simulink model "GameModel"  (R2024a)
settings: Solver=VariableStepAuto  StartTime=0.0  StopTime=inf  MaxStep=0.02  RelTol=1e-3
model workspace (MAT data in the model file):
  g = 9.81
undefined symbols (not defined in the file or in its folder): CR, LF
libraries: simulink x8, instrumentseriallib x2
settings Model: Creator=Admin  LastModifiedBy=Michael Scopchanov

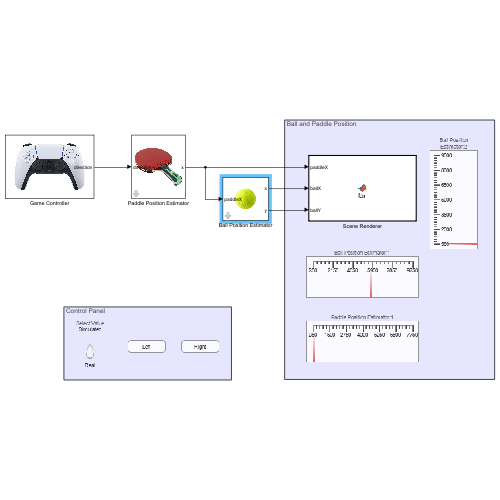
[thumbnail: Simulink's stored preview of the top-level diagram]
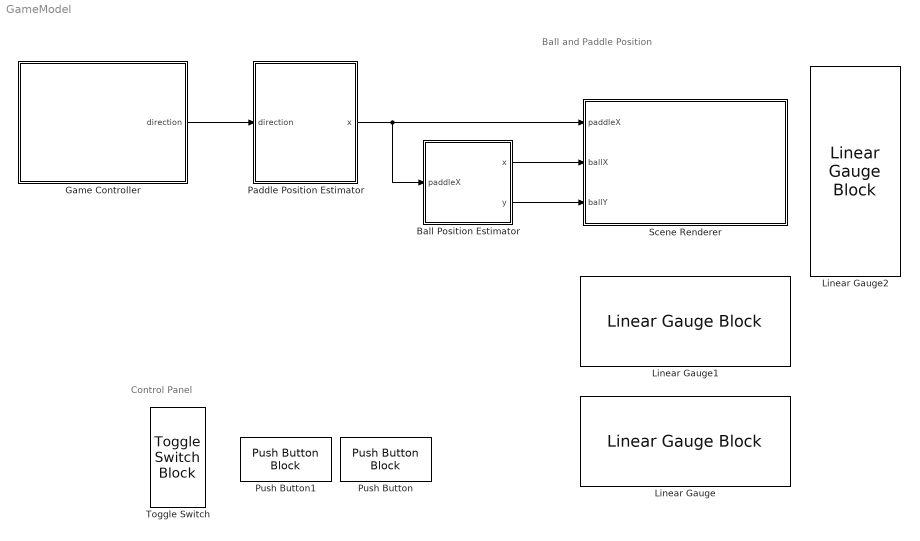
== system GameModel ==
  note: Ball and Paddle Position
  note: Control Panel
  Ball Position Estimator : Subsystem  mask{m=0.05, x0=4875, y0=4000, vn=10000}
      mask prompts: m "Mass [kg]"; x0 "Initial Position x [m]"; y0 "Initial Position y [m]"; vn "Nominal velocity [m/s]"
      mask Display: image('ball.png', [20,20,20,20,100,100]);
  Game Controller : Subsystem
      mask Display: image('controller.png', [10,10,10,10,100,100]);
  Linear Gauge : LinearGaugeBlock  ScaleMin=250  ScaleMax=7750
  Linear Gauge1 : LinearGaugeBlock  ScaleMin=250  ScaleMax=9750
  Linear Gauge2 : LinearGaugeBlock  ScaleMin=500  ScaleMax=9500
  Paddle Position Estimator : Subsystem  mask(Paddle Position Estimator){vn=15000, x0=4000, xmin=250, xmax=7750}
      mask prompts: vn "Nominal velocity [m/s]"; x0 "Initial position [m]"; xmin "Minimal position [m]"; xmax "Maximum position [m]"
      mask Display: image('paddle.jpg');
  Push Button : PushButtonBlock  ButtonText=Right  OnValue=0  OffValue=1.000000
  Push Button1 : PushButtonBlock  ButtonText=Left  OnValue=0  OffValue=1.000000
  Scene Renderer : MATLAB Function  InitFcn=handles = setupGraphics();  TreatAsAtomicUnit=on
  Toggle Switch : ToggleSwitchBlock
      settings: Values={{'Real', 'Simulated'}, [0 1]}
  wires:
  Game Controller/1(direction) -> Paddle Position Estimator/1(direction)
  Ball Position Estimator/1(x) -> Scene Renderer/2(ballX)
  Ball Position Estimator/2(y) -> Scene Renderer/3(ballY)
  Paddle Position Estimator/1(x) -> Ball Position Estimator/1(paddleX), Scene Renderer/1(paddleX)

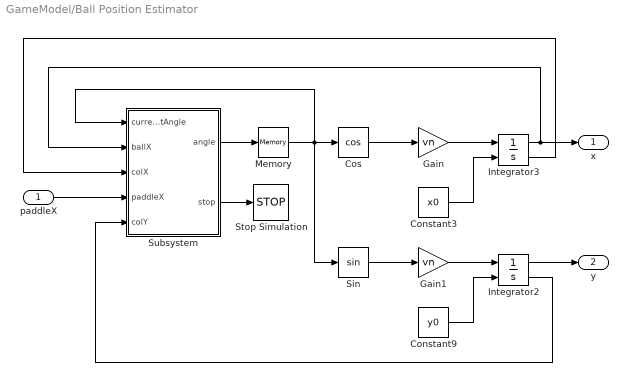
== system GameModel/Ball Position Estimator ==
  paddleX : Inport
  Constant3 : Constant  Value=x0
  Constant9 : Constant  Value=y0
  Cos : Trigonometry  Operator=cos
  Gain : Gain  Gain=vn
  Gain1 : Gain  Gain=vn
  Integrator2 : Integrator  InitialConditionSource=external  LimitOutput=on  UpperSaturationLimit=9500  LowerSaturationLimit=500  ShowSaturationPort=on
  Integrator3 : Integrator  InitialConditionSource=external  LimitOutput=on  UpperSaturationLimit=9500  LowerSaturationLimit=250  ShowSaturationPort=on
  Memory : Memory  InitialCondition=pi/3
  Sin : Trigonometry
  Stop Simulation : Stop
  Subsystem : Subsystem
  x : Outport
  y : Outport  Port=2
  wires:
  Integrator3/1 -> x/1, Subsystem/2(ballX)
  Constant3/1 -> Integrator3/2
  Integrator3/2 -> Subsystem/3(colX)
  Integrator2/2 -> Subsystem/5(colY)
  Constant9/1 -> Integrator2/2
  Integrator2/1 -> y/1
  Sin/1 -> Gain1/1
  Cos/1 -> Gain/1
  Memory/1 -> Subsystem/1(currentAngle), Sin/1, Cos/1
  Subsystem/1(angle) -> Memory/1
  paddleX/1 -> Subsystem/4(paddleX)
  Gain/1 -> Integrator3/1
  Gain1/1 -> Integrator2/1
  Subsystem/2(stop) -> Stop Simulation/1

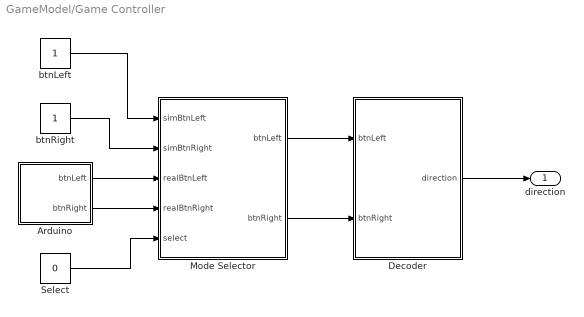
== system GameModel/Game Controller ==
  Arduino : Subsystem
      mask Display: image('arduino.jpg');
  Decoder : Subsystem
  Mode Selector : Subsystem
  Select : Constant  Value=0
  btnLeft : Constant
  btnRight : Constant
  direction : Outport
  wires:
  Arduino/2(btnRight) -> Mode Selector/4(realBtnRight)
  btnRight/1 -> Mode Selector/2(simBtnRight)
  Mode Selector/1(btnLeft) -> Decoder/1(btnLeft)
  Mode Selector/2(btnRight) -> Decoder/2(btnRight)
  btnLeft/1 -> Mode Selector/1(simBtnLeft)
  Decoder/1(direction) -> direction/1
  Select/1 -> Mode Selector/5(select)
  Arduino/1(btnLeft) -> Mode Selector/3(realBtnLeft)

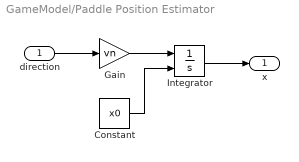
== system GameModel/Paddle Position Estimator ==
  direction : Inport
  Constant : Constant  Value=x0
  Gain : Gain  Gain=vn
  Integrator : Integrator  InitialConditionSource=external  LimitOutput=on  UpperSaturationLimit=xmax  LowerSaturationLimit=xmin
  x : Outport
  wires:
  direction/1 -> Gain/1
  Gain/1 -> Integrator/1
  Integrator/1 -> x/1
  Constant/1 -> Integrator/2

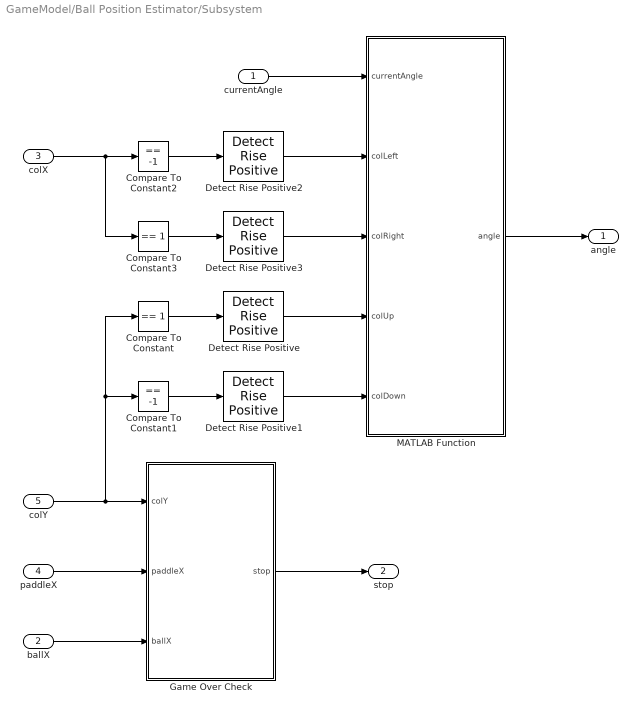
== system GameModel/Ball Position Estimator/Subsystem ==
  currentAngle : Inport
  ballX : Inport  Port=2
  colX : Inport  Port=3
  paddleX : Inport  Port=4
  colY : Inport  Port=5
  Compare To Constant : simulink/Logic and Bit Operations/Compare To Constant  relop===  const=1  OutDataTypeStr=boolean
  Compare To Constant1 : simulink/Logic and Bit Operations/Compare To Constant  relop===  const=-1  OutDataTypeStr=boolean
  Compare To Constant2 : simulink/Logic and Bit Operations/Compare To Constant  relop===  const=-1  OutDataTypeStr=boolean
  Compare To Constant3 : simulink/Logic and Bit Operations/Compare To Constant  relop===  const=1  OutDataTypeStr=boolean
  Detect Rise Positive{,1..3} (4 alike) : simulink/Logic and Bit Operations/Detect Rise Positive  vinit=0  OutDataTypeStr=boolean
  Game Over Check : MATLAB Function  TreatAsAtomicUnit=on
  MATLAB Function : MATLAB Function  TreatAsAtomicUnit=on
  angle : Outport
  stop : Outport  Port=2
  wires:
  MATLAB Function/1(angle) -> angle/1
  colY/1 -> Game Over Check/1(colY), Compare To Constant/1, Compare To Constant1/1
  paddleX/1 -> Game Over Check/2(paddleX)
  ballX/1 -> Game Over Check/3(ballX)
  Game Over Check/1(stop) -> stop/1
  currentAngle/1 -> MATLAB Function/1(currentAngle)
  colX/1 -> Compare To Constant3/1, Compare To Constant2/1
  Compare To Constant/1 -> Detect Rise Positive/1
  Detect Rise Positive/1 -> MATLAB Function/4(colUp)
  Compare To Constant1/1 -> Detect Rise Positive1/1
  Detect Rise Positive1/1 -> MATLAB Function/5(colDown)
  Compare To Constant2/1 -> Detect Rise Positive2/1
  Detect Rise Positive2/1 -> MATLAB Function/2(colLeft)
  Compare To Constant3/1 -> Detect Rise Positive3/1
  Detect Rise Positive3/1 -> MATLAB Function/3(colRight)

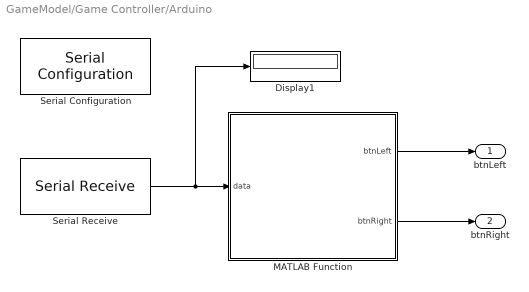
== system GameModel/Game Controller/Arduino ==
  Display1 : Display
  MATLAB Function : MATLAB Function  TreatAsAtomicUnit=on
  Serial Configuration : instrumentseriallib/Serial Configuration  Priority=-200000  PortSel=COM3  Port=COM3  ComPort=COM3  BaudRate=19200  DataBits=8  Parity=none  StopBits=1  ByteOrder=little-endian  FlowControl=none  Timeout=10  SimulateUsing=Interpreted execution  BlockInModel=on  aMode=1
  Serial Receive : instrumentseriallib/Serial Receive  Priority=1  PortSel=COM3  Port=COM3  ComPort=COM3  DataType=uint8  SaveDataType=uint8  ToggleHeader=off  Header=[]  ToggleDataSize=on  DataSize=[1 1]  ToggleTerminator=off  Terminator=CR/LF ('\r\n')  CustomTerminator=[]  InputFormat=Column major  EnableBlockingMode=on  ActionDataUnavailable=Output custom value  ActionWhenDataUnavailable=Output custom value  CustomValue=0  SampleTime=0.01  SimulateUsing=Interpreted execution  BlockInModel=on  aMode=1
  btnLeft : Outport
  btnRight : Outport  Port=2
  wires:
  MATLAB Function/1(btnLeft) -> btnLeft/1
  MATLAB Function/2(btnRight) -> btnRight/1
  Serial Receive/1 -> Display1/1, MATLAB Function/1(data)

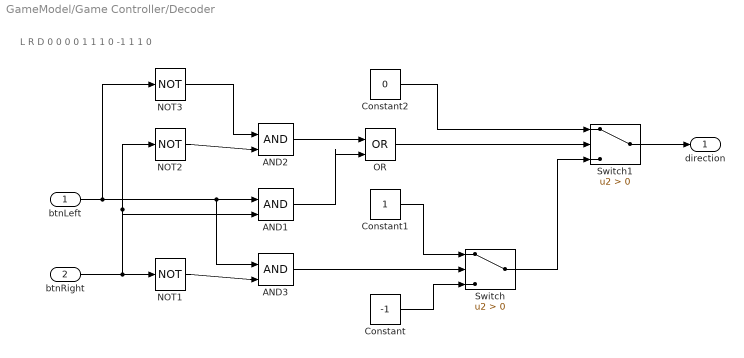
== system GameModel/Game Controller/Decoder ==
  note: L
      | R
      | D
      |
      | 0
      | 0
      | 0
      |
      | 0
      | 1
      | 1
      |
      | 1
      | 0
      | -1
      |
      | 1
      | 1
      | 0
  btnLeft : Inport
  btnRight : Inport  Port=2
  AND1 : Logic  IconShape=distinctive  AllPortsSameDT=off  OutDataTypeStr=boolean
  AND2 : Logic  IconShape=distinctive  AllPortsSameDT=off  OutDataTypeStr=boolean
  AND3 : Logic  IconShape=distinctive  AllPortsSameDT=off  OutDataTypeStr=boolean
  Constant : Constant  Value=-1
  Constant1 : Constant
  Constant2 : Constant  Value=0
  NOT1 : Logic  Operator=NOT  IconShape=distinctive  AllPortsSameDT=off  OutDataTypeStr=boolean
  NOT2 : Logic  Operator=NOT  IconShape=distinctive  AllPortsSameDT=off  OutDataTypeStr=boolean
  NOT3 : Logic  Operator=NOT  IconShape=distinctive  AllPortsSameDT=off  OutDataTypeStr=boolean
  OR : Logic  Operator=OR  IconShape=distinctive  AllPortsSameDT=off  OutDataTypeStr=boolean
  Switch : Switch  Criteria=u2 > Threshold  SaturateOnIntegerOverflow=off  InputSameDT=off
  Switch1 : Switch  Criteria=u2 > Threshold  SaturateOnIntegerOverflow=off  InputSameDT=off
  direction : Outport
  wires:
  Constant1/1 -> Switch/1
  AND3/1 -> Switch/2
  Constant/1 -> Switch/3
  Constant2/1 -> Switch1/1
  NOT3/1 -> AND2/1
  NOT1/1 -> AND3/2
  btnRight/1 -> NOT1/1, NOT2/1, AND1/2
  OR/1 -> Switch1/2
  btnLeft/1 -> NOT3/1, AND3/1, AND1/1
  AND2/1 -> OR/1
  Switch/1 -> Switch1/3
  AND1/1 -> OR/2
  NOT2/1 -> AND2/2
  Switch1/1 -> direction/1

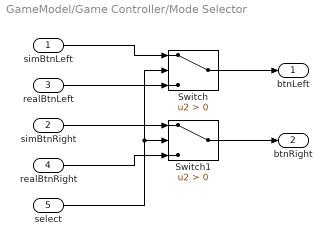
== system GameModel/Game Controller/Mode Selector ==
  simBtnLeft : Inport
  simBtnRight : Inport  Port=2
  realBtnLeft : Inport  Port=3
  realBtnRight : Inport  Port=4
  select : Inport  Port=5
  Switch : Switch  Criteria=u2 > Threshold  SaturateOnIntegerOverflow=off  InputSameDT=off
  Switch1 : Switch  Criteria=u2 > Threshold  SaturateOnIntegerOverflow=off  InputSameDT=off
  btnLeft : Outport
  btnRight : Outport  Port=2
  wires:
  Switch/1 -> btnLeft/1
  Switch1/1 -> btnRight/1
  simBtnLeft/1 -> Switch/1
  simBtnRight/1 -> Switch1/1
  realBtnLeft/1 -> Switch/3
  realBtnRight/1 -> Switch1/3
  select/1 -> Switch/2, Switch1/2

== matlab function GameModel/Ball Position Estimator/Subsystem/Game Over Check ==
  data: colY input; paddleX input; stop output; ballX input
function stop = fcn(colY, paddleX, ballX)

stop = colY == -1 && (ballX + 250 < paddleX || ballX > paddleX + 2000);

== matlab function GameModel/Scene Renderer ==
  data: paddleX input; ballX input; ballY input
function fcn(paddleX, ballX, ballY)

coder.extrinsic('evalin', 'plot')

paddleHandle = evalin('base', 'handles.paddle');
ballHandle = evalin('base', 'handles.ball');

set(paddleHandle, 'Position', [paddleX 250 2000 250]);
set(ballHandle, 'Position', [ballX ballY 250 250]);

drawnow('limitrate')
% pause(0.001)

== matlab function GameModel/Ball Position Estimator/Subsystem/MATLAB Function ==
  data: currentAngle input; colLeft input; colRight input; angle output; colUp input; colDown input
function angle = fcn(currentAngle, colLeft, colRight, colUp, colDown)

angle = currentAngle;

if colLeft
    angle = -currentAngle + pi;
end

if colRight
    angle = -currentAngle + pi;
end

if colUp
    angle = -currentAngle;
end

if colDown
    angle = -currentAngle;
end


rad2deg(angle)

% -1.05*pi/2

== matlab function GameModel/Game Controller/Arduino/MATLAB Function ==
  data: data input; btnLeft output; btnRight output
function [btnLeft, btnRight] = parseSerialData(data)
    % Konvertiere das Daten-Array in einen String
    str = char(data');

    % Entferne Zeilenumbruch und Leerzeichen
    str = strtrim(str);

    % Initialisiere die Ausgänge
    btnLeft = 0;
    btnRight = 0;

    % Überprüfen Sie die empfangenen Daten und setzen Sie die Schaltflächen
    switch str
        case 'M'
            btnLeft = 1;
            btnRight = 0;
        case 'N'
            btnLeft = 0;
            btnRight = 1;
        case 'O'
            btnLeft = 1;
            btnRight = 1;
        case 'P'
            btnLeft = 0;
            btnRight = 0;
    end

    display(str)
end
